simulink model "new_open_loop_DAD 2022"  (R2024a)
settings: Solver=VariableStepAuto  StartTime=0.0  StopTime=0.01  RelTol=1e-3
libraries: spsMosfetLib x8, spsVoltageMeasurementLib x4, spsLinearTransformerLib x1, spsCurrentMeasurementLib x1, spsDCVoltageSourceLib x1, spsParallelRLCBranchLib x1, spsSeriesRLCBranchLib x1, spspowerguiLib x1
settings Model: Creator=Lenovo  LastModifiedBy=Lenovo

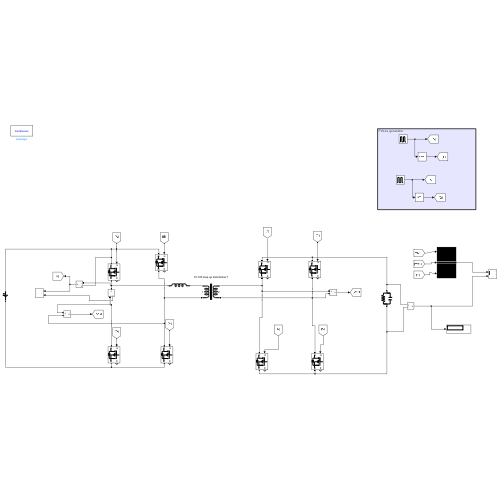
[thumbnail: Simulink's stored preview of the top-level diagram]
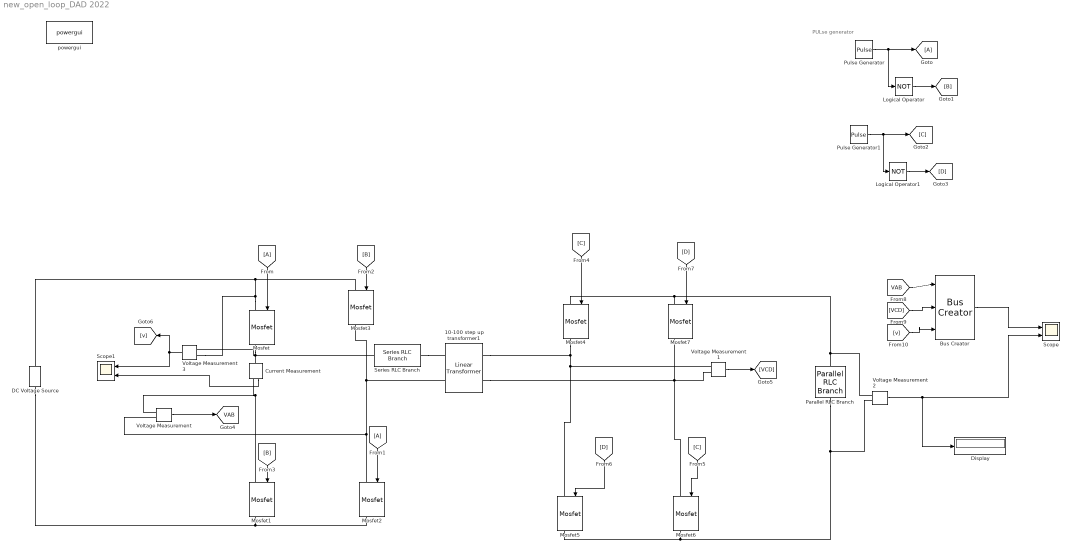
== system new_open_loop_DAD 2022 ==
  note: PULse generator
  10-100 step up transformer1 : spsLinearTransformerLib/Linear Transformer  UNITS=pu  NominalPower=[ 2.5e3 500e3 ]  winding1="[ 100 0  0 ]"  winding2="[ 700  0  0 ]"  ThreeWindings=off  winding3=[ 315e3 0.002 0.08 ]  RmLm="[ 1e6  1e6 ]"  Measurements=None  DataType=off
  Bus Creator : BusCreator  Inputs=3
  Current Measurement : spsCurrentMeasurementLib/Current Measurement  PhasorSimulation=off  OutputType=Complex  PSBequivalent=0
  DC Voltage Source : spsDCVoltageSourceLib/DC Voltage Source  Amplitude=400  Measurements=None
  Display : Display
  From : From
  From1 : From
  Goto : Goto
  Logical Operator : Logic  Operator=NOT  AllPortsSameDT=off  OutDataTypeStr=boolean
  Logical Operator1 : Logic  Operator=NOT  AllPortsSameDT=off  OutDataTypeStr=boolean
  Mosfet{,1..7} (8 alike) : spsMosfetLib/Mosfet  Ron=0.1  Lon=0  Rd=0.01  Vfd=0  IC=0  Rs=1e5  Cs=inf  Measurements=on
  Parallel RLC Branch : spsParallelRLCBranchLib/Parallel RLC Branch  LConnTagsString=a  RConnTagsString=__new0  BranchType=RC  Resistance=73  Inductance=1e-3  SetiL0=off  InitialCurrent=0  Capacitance=100e-6  Setx0=off  InitialVoltage=0  Measurements=None
  Pulse Generator : DiscretePulseGenerator  PulseType=Time based  Period=1/500e3  PulseWidth=50  PhaseDelay=(63/360)*((1/500e3))
  Pulse Generator1 : DiscretePulseGenerator  PulseType=Time based  Period=1/500e3  PulseWidth=50  PhaseDelay=(63/360)*(1/(500e3))
  Scope : Scope  NumInputPorts=2
  Scope1 : Scope  NumInputPorts=2
  Series RLC Branch : spsSeriesRLCBranchLib/Series RLC Branch  LConnTagsString=__new0  RConnTagsString=__new0  BranchType=L  Resistance=1  Inductance=0.3e-6  SetiL0=off  InitialCurrent=0  Capacitance=1e-6  Setx0=off  InitialVoltage=0  Measurements=None
  Voltage Measurement{,1..3} (4 alike) : spsVoltageMeasurementLib/Voltage Measurement  PhasorSimulation=off  OutputType=Complex  PSBequivalent=0
  powergui : spspowerguiLib/powergui  Priority=1  SimulationMode=Continuous  SampleTime=50e-6  frequency=60  Iterations=50  frequencyindice=0  Pbase=100e6  ErrMax=1e-4  UnitsV=kV  UnitsW=MW  buscounter=0  FunctionMessages=off  echomessages=off  EnableUseOfTLC=off  CurrentSourceSwitches=off  DisableSnubberDevices=off  DisableRonSwitches=off  DisableVfSwitches=off  DisplayEquations=off  AutomaticDiscreteSolvers=off  SolverType=Tustin/Backward Euler (TBE)  Interpol=off  ExternalGateDelay=off  methode=off  Ts=100  x0status=blocks  SPID=on  SwTol=0  HookPort=off  NonlinearTolerance=1e-4  nMaxIteration=100  ContinueOnMaxIteration=off  RestoreLinks=warning  ResistiveCurrentMeasurement=off  Frange=[0:2:500]  Ylog=off  Xlog=on  ShowGrid=off  save=off  variable=ZData  structure=0  ZoomFFT=off  StartTime=0.0  cycles=1  DisplayStyle=1  fundamental=60  FreqAxis=off  MaxFrequency=1000  frequencyindicesteady=1  RmsSteady=1  display=off
  tag scope: VAB=global
  wires:
  Voltage Measurement3/1 -> Scope1/1, [v]
  Current Measurement/1 -> Scope1/2
  [B] -> Mosfet1/1
  [B] -> Mosfet3/1
  [D] -> Mosfet5/1
  [VCD] -> Bus Creator/2
  From1/1 -> Mosfet2/1
  From/1 -> Mosfet/1
  [D] -> Mosfet7/1
  [C] -> Mosfet4/1
  [C] -> Mosfet6/1
  [VAB] -> Bus Creator/1
  Logical Operator/1 -> [B]
  Voltage Measurement1/1 -> [VCD]
  Pulse Generator/1 -> Logical Operator/1, Goto/1
  Bus Creator/1 -> Scope/1
  Pulse Generator1/1 -> [C], Logical Operator1/1
  [v] -> Bus Creator/3
  Logical Operator1/1 -> [D]
  Voltage Measurement/1 -> [VAB]
  Voltage Measurement2/1 -> Display/1, Scope/2
  connections:
  Voltage Measurement/LConn1 -- Current Measurement/RConn1 -- Mosfet1/LConn1
  Mosfet5/RConn1 -- Mosfet6/RConn1 -- Parallel RLC Branch/RConn1 -- Voltage Measurement2/LConn2
  Mosfet4/RConn1 -- Voltage Measurement1/LConn1 -- Mosfet5/LConn1 -- 10-100 step up transformer1/RConn1
  Parallel RLC Branch/LConn1 -- Mosfet4/LConn1 -- Mosfet7/LConn1 -- Voltage Measurement2/LConn1
  Mosfet3/RConn1 -- Voltage Measurement/LConn2 -- Mosfet2/LConn1 -- 10-100 step up transformer1/LConn2
  Mosfet1/RConn1 -- DC Voltage Source/LConn1 -- Mosfet2/RConn1
  Mosfet/LConn1 -- Mosfet3/LConn1 -- DC Voltage Source/RConn1 -- Voltage Measurement3/LConn1
  10-100 step up transformer1/RConn2 -- Mosfet7/RConn1 -- Voltage Measurement1/LConn2 -- Mosfet6/LConn1
  Mosfet/RConn1 -- Current Measurement/LConn1 -- Series RLC Branch/LConn1 -- Voltage Measurement3/LConn2
  Series RLC Branch/RConn1 -- 10-100 step up transformer1/LConn1
